simulink library "CM010A_GmT1xxMcuCfg_ModelLibrary"  (Simulink 8.2)
settings: Solver=ode45  StartTime=0.0  StopTime=10.0  RelTol=1e-3
undefined symbols (not defined in the file): ADC0CFGANDUSE_ADCSCAGFAC_VOLTPERCNT_F32
libraries: CM010A_GmT1xxMcuCfg_ModelLibrary x1
settings Model: Creator=nz3zln  LastModifiedBy=nz3zln

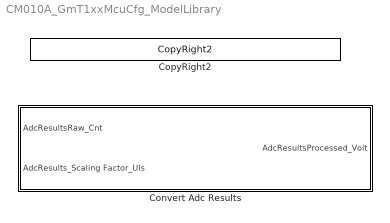
== system CM010A_GmT1xxMcuCfg_ModelLibrary ==
  Convert Adc Results : Subsystem  TreatAsAtomicUnit=on
  CopyRight2 : CM010A_GmT1xxMcuCfg_ModelLibrary/Convert Adc Results/CopyRight2  Description=|  none=on
      | Copyright info block.                                               
      |                                                                     
      | Place copyright information at the top of every subsystem in design.

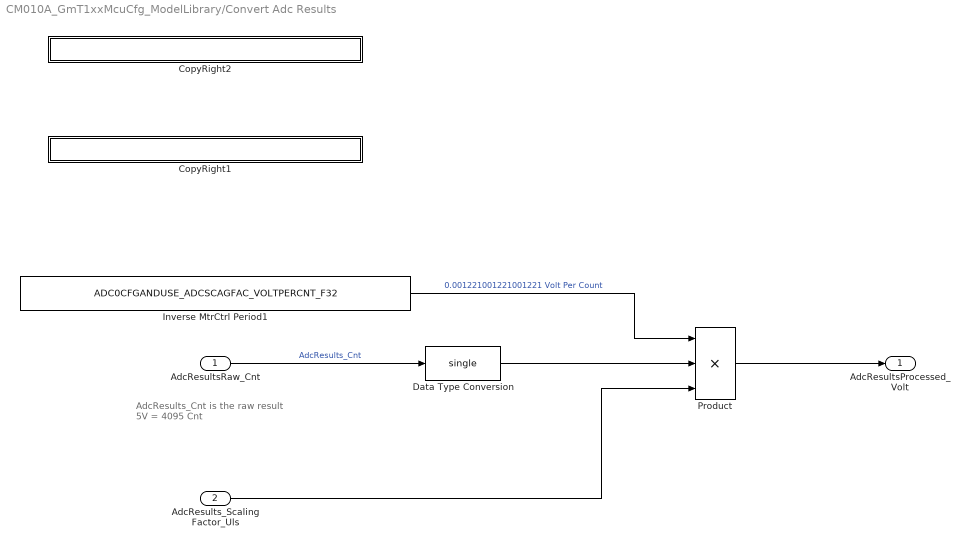
== system CM010A_GmT1xxMcuCfg_ModelLibrary/Convert Adc Results ==
  note: AdcResults_Cnt is the raw result
      |
      | 5V = 4095 Cnt
  AdcResultsRaw_Cnt : Inport
  AdcResults_Scaling Factor_Uls : Inport  Port=2  OutDataTypeStr=single
  CopyRight1 : Subsystem  Description=|  mask(Copyright Information){none=on}
      | Copyright info block.                                               
      |                                                                     
      | Place copyright information at the top of every subsystem in design.
      mask prompts: none "No parameters"
      mask help: Place copyright information at the top of every subsystem in design.
      mask Display:
      | NxtrConf = 'Nexteer Confidential';
      | 
      | sys = bdroot; %handle for the current model ("system")
      | first = get_param(sys,'Created');
      | first = first(end-3:end);  %year is last four digits
      | 
      | last = get_param(sys,'LastModifiedDate');
      | if isempty(last)
      |     last = datestr(now,'yyyy');
      | else
      |     last = last(end-3:end);
      | end
      | 
      | if strcmp(first,last)
      |     fprintf('%s -- Copyright %s Nexteer',NxtrConf,first)
      | else
      |     fprintf('%s -- %s%s- %s Nexteer',NxtrConf,char(169),first,last)
      | end
  CopyRight2 : Subsystem  Description=|  mask(Copyright Information){none=on}
      | Copyright info block.                                               
      |                                                                     
      | Place copyright information at the top of every subsystem in design.
      mask prompts: none "No parameters"
      mask help: Place copyright information at the top of every subsystem in design.
      mask Display:
      | NxtrConf = 'Nexteer Confidential';
      | 
      | sys = bdroot; %handle for the current model ("system")
      | first = get_param(sys,'Created');
      | if(isempty(first))
      |     first = datestr(now,'yyyy');
      | else
      |     first = first(end-3:end);  %year is last four digits
      | end
      | 
      | last = get_param(sys,'LastModifiedDate');
      | if isempty(last)
      |     last = datestr(now,'yyyy');
      | else
      |     last = last(end-3:end);
      | end
      | 
      | if strcmp(first,last)
      |     fprintf('%s -- Copyright %s Nexteer',NxtrConf,first)
      | else
      |     fprintf('%s -- %s%s- %s Nexteer',NxtrConf,char(169),first,last)
      | end
  Data Type Conversion : DataTypeConversion  OutDataTypeStr=single
  Inverse MtrCtrl Period1 : Constant  Value=ADC0CFGANDUSE_ADCSCAGFAC_VOLTPERCNT_F32  OutDataTypeStr=single
  Product : Product  Inputs=3  OutDataTypeStr=single
  AdcResultsProcessed_Volt : Outport  OutDataTypeStr=single
  wires:
  AdcResultsRaw_Cnt/1 -> Data Type Conversion/1  "AdcResults_Cnt"
  Inverse MtrCtrl Period1/1 -> Product/1  "0.001221001221001221 Volt Per Count"
  Data Type Conversion/1 -> Product/2
  AdcResults_Scaling Factor_Uls/1 -> Product/3
  Product/1 -> AdcResultsProcessed_Volt/1

== system CM010A_GmT1xxMcuCfg_ModelLibrary/Convert Adc Results/CopyRight1 ==

== system CM010A_GmT1xxMcuCfg_ModelLibrary/Convert Adc Results/CopyRight2 ==
